simulink model "3_pole_simulink"  (R2023b)
settings: Solver=VariableStepAuto  StartTime=0.0  StopTime=20  RelTol=1e-3
settings Model: Creator=mampane  LastModifiedBy=dkim4

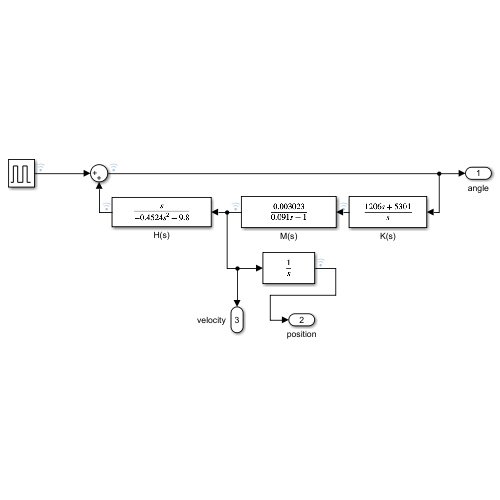
[thumbnail: Simulink's stored preview of the top-level diagram]
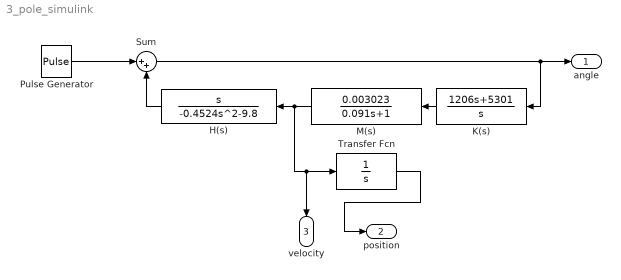
== system 3_pole_simulink ==
  H(s) : TransferFcn  Numerator=[1 0]  Denominator=[-0.4524 0 -9.8]
  K(s) : TransferFcn  Numerator=[1206 5301]  Denominator=[1 0]
  M(s) : TransferFcn  Numerator=[0.003023]  Denominator=[0.091 1]
  Pulse Generator : DiscretePulseGenerator  PulseType=Time based  Amplitude=1/36  Period=10  PulseWidth=0.1
  Sum : Sum  Inputs=|++
  Transfer Fcn : TransferFcn  Denominator=[1 0]
  angle : Outport
  position : Outport  Port=2
  velocity : Outport  Port=3
  wires:
  H(s)/1 -> Sum/2
  Pulse Generator/1 -> Sum/1
  M(s)/1 -> velocity/1, Transfer Fcn/1, H(s)/1
  Sum/1 -> angle/1, K(s)/1
  Transfer Fcn/1 -> position/1
  K(s)/1 -> M(s)/1
